simulink model "DT_Model_Matching_Desired_with_Controller"  (R2015a)
settings: Solver=FixedStepDiscrete  StartTime=0.0  StopTime=Tf  FixedStep=Ts  MaxStep=1e-5  RelTol=1e-4
values from neighbouring files (symbols this model uses):
  Ac = (abs(den_Gc) > tol*ones(1,length(den_Gc))).*den_Gc    [DT_model_matching_driver.m]
  Bc = (abs(num_Gc) > tol*ones(1,length(num_Gc))).*num_Gc    [DT_model_matching_driver.m]
  Ts = 0.05    [wheel_parameters.m]
undefined symbols (not defined in the file or in its folder): den_Gp, num_Gp
settings Model: Creator=throne  LastModifiedBy=throne
settings DataIOCC: SignalLoggingSaveFormat=ModelDataLogs  SignalLoggingName=sigsOut
settings OptimizationCC: ExpressionDepthLimit=2147483647
settings DebuggingCC: SaveWithParameterizedLinksMsg=none  UnderspecifiedInitializationDetection=Classic  MergeDetectMultiDrivingBlocksExec=none  SignalResolutionControl=TryResolveAllWithWarning  MultiTaskDSMMsg=warning  MultiTaskCondExecSysMsg=none  StateNameClashWarn=warning
settings HardwareCC: TargetUnknown=on
settings GRTTargetCC: CombineOutputUpdateFcns=off  GRTInterface=on

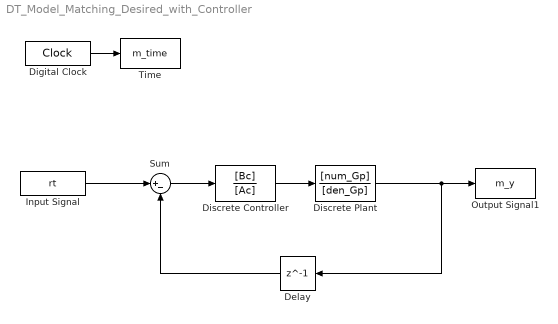
== system DT_Model_Matching_Desired_with_Controller ==
  Delay : Delay  DelayLength=1  InitialCondition=0  SampleTime=Ts
  Digital Clock : DigitalClock  SampleTime=Ts
  Discrete Controller : DiscreteTransferFcn  Numerator=[Bc]  Denominator=[Ac]  SampleTime=Ts
  Discrete Plant : DiscreteTransferFcn  Numerator=[num_Gp]  Denominator=[den_Gp]  SampleTime=Ts
  "Input Signal " : FromWorkspace  VariableName=rt  SampleTime=Ts
  Output Signal1 : ToWorkspace  VariableName=m_y  SampleTime=-1
  Sum : Sum  Inputs=|+-
  Time : ToWorkspace  VariableName=m_time  SampleTime=-1
  wires:
  Digital Clock/1 -> Time/1
  "Input Signal "/1 -> Sum/1
  Discrete Plant/1 -> Delay/1, Output Signal1/1
  Discrete Controller/1 -> Discrete Plant/1
  Delay/1 -> Sum/2
  Sum/1 -> Discrete Controller/1
